simulink model "DiscreteSystem"  (R2026a)
settings: Solver=VariableStepAuto
StartFcn:
  | learning.simulink.modelCallbacks.startFunction(gcs);
StopFcn:
  | learning.simulink.modelCallbacks.stopFunction(gcs);
model workspace (MAT data in the model file):
  courseObject.course = 'simulink'
  courseObject.chapter = 9
  courseObject.lesson = 1
  courseObject.section = 1
  courseObject.task = 1
  t_ans = [0; 0.2; 0.4; 0.6; 0.8; 1; 1.2; 1.4; 1.6; 1.8; 2; 2.2; 2.4; 2.6; 2.8; 3; 3.2; 3.4; 3.6; 3.8; 4; 4.2; 4.4; 4.6; 4.8; 5; 5.2; 5.4; 5.6; 5.8; 6; 6.2; 6.4; 6.6; 6.8; 7; 7.2; 7.4; 7.6; 7.8; 8; 8.2; 8.4; 8.6; 8.8; 9; 9.2; 9.4; 9.6; 9.8; 10]
  y_ans2 = [0; 0; 0.198669330795; 0.389418342309; 0.564642473395; 0.7173560909; 0.841470984808; 0.932039085967; 0.985449729988; 0.999573603042; 0.973847630878; 0.909297426826; 0.80849640382; 0.675463180551; 0.515501371821; 0.334988150156; 0.14112000806; -0.0583741434276; -0.255541102027; -0.442520443295; -0.611857890943; -0.756802495308; -0.871575772414; -0.95160207389; -0.993691003633; -0.996164608836; -0.958924274663; -0.88345465572; -0.772764487556; -0.631266637872; -0.464602179414; -0.279415498199; -0.0830894028175; 0.11654920485; 0.311541363513; 0.494113351139; 0.656986598719; 0.793667863849; 0.898708095812; 0.967919672031; 0.998543345375; 0.989358246623; 0.94073055668; 0.854598908088; 0.734397097874; 0.584917192892; 0.412118485242; 0.2228899141; 0.0247754254534; -0.174326781223; -0.366479129252]
libraries: signalChecks x1
CloseFcn:
  | learning.simulink.cleanupOnlineTraining;learning.simulink.Application.getInstance().dduxLogMatlabEvent("ModelClosed");
Description:
  | TrainingCourseModel
settings Model: Creator=PC  LastModifiedBy=PC

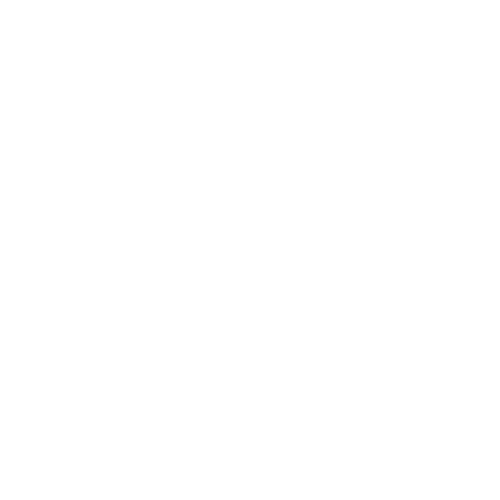
[thumbnail: Simulink's stored preview of the top-level diagram]
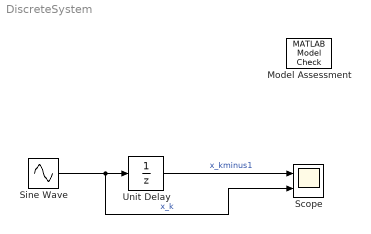
== system DiscreteSystem ==
  Model Assessment : signalChecks/MATLAB Model Check  mlfunc='grader_interaction1_task5'  lesson=0  task=5  pass=-1
      settings: AttributesFormatString=|
      | No input required
      | for this task
  Scope : Scope  NumInputPorts=2
  Sine Wave : Sin  SampleTime=0.25
  Unit Delay : UnitDelay  SampleTime=0.5
  wires:
  Sine Wave/1 -> Scope/2, Unit Delay/1  "x_k"
  Unit Delay/1 -> Scope/1  "x_kminus1"
